simulink model "main"  (R2023a)
settings: Solver=VariableStepAuto  StartTime=0.0  StopTime=1  RelTol=1e-9  AbsTol=1e-9  EnableMultiTasking=on
values from neighbouring files (symbols this model uses):
  a_el = [r_ej,h_ej,r_ej]    [data.m]    (also in fo_python_to_matlab.m = [ax,ay,az])
  akt_GH = rand(1,13)*1    [inverse_dynamics.m]    (also in odvozeni_svaly.m = sym('akt_GH',[1 N_GH]))
  akt_ST = rand(1,13)*1    [inverse_dynamics.m]    (also in odvozeni_svaly.m = sym('akt_ST',[1 N_ST]))
  ax = r_ej    (= 0.088)    [data.m]
  ay = h_ej    (= 0.15)    [data.m]
  az = r_ej    (= 0.088)    [data.m]
  ccom = [-0.0110972, 0.00637508, 0.0541825]    [data.m]    (also in fo_python_to_matlab.m = [ccomx, ccomy, ccomz]; mm_python_to_matlab.m = [ccomx, ccomy, ccomz])
  cI = [5.75482e-05, 6.05521e-05, 1.05345e-05,-1.27405e-05, 1.65861e-05, 4.50136e-06]    [data.m]    (also in mm_python_to_matlab.m = [cixx, ciyy, cizz, cixy, ciyz, cizx])
  cont1 = [-0.083529 -0.01368 -0.098954]-scom    [data.m]    (also in fo_python_to_matlab.m = [x_cont1,y_cont1,z_cont1])
  cont2 = [-0.105456 -0.125076 -0.075251]-scom    [data.m]    (also in fo_python_to_matlab.m = [x_cont2,y_cont2,z_cont2])
  cont_params = [k_contact, eps]    [data.m]    (also in fo_python_to_matlab.m)
  Glenohumeral_F0M = str2double(table2array(GH(:,2)))'    [data.m]
  Glenohumeral_l0 = str2double(table2array(GH(:,3)))'    [data.m]
  h_ej = 0.15    [data.m]
  hcom = [0.000389382, -0.116338, -0.00231072]    [data.m]    (also in fo_python_to_matlab.m = [hcomx, hcomy, hcomz]; mm_python_to_matlab.m = [hcomx, hcomy, hcomz])
  hI = [0.00326632, 4.34807e-05, 0.00325004,-0.000136456, -1.30958e-06, -1.14964e-05]    [data.m]    (also in mm_python_to_matlab.m = [hixx, hiyy, hizz, hixy, hiyz, hizx])
  initialConditions = zeros(1,18)    [inverse_dynamics.m]
  k_contact = 0    [data.m]
  m = [0.0370005,0.12759,0.26363]    [data.m]    (also in fo_python_to_matlab.m = [c_m,s_m,h_m]; mm_python_to_matlab.m = [c_m,s_m,h_m])
  m_el = [x_ej,y_ej,z_ej]    [data.m]    (also in fo_python_to_matlab.m = [mx, my, mz])
  mx = x_ej    (= -0.03)    [data.m]
  my = y_ej    (= -0.1)    [data.m]
  mz = z_ej    (= 0.05)    [data.m]
  p = [c,k,g]    [data.m]    (also in fo_python_to_matlab.m)
  r_ej = 0.088    [data.m]
  Scapulothoracic_F0M = str2double(table2array(ST(:,2)))'    [data.m]
  Scapulothoracic_l0 = str2double(table2array(ST(:,3)))'    [data.m]
  scom = [-0.0512948, -0.0367122, -0.0430756]    [data.m]    (also in fo_python_to_matlab.m = [scomx, scomy, scomz]; mm_python_to_matlab.m = [scomx, scomy, scomz])
  sI = [0.00020065, 0.000202939, 0.000227237,-4.55661e-05, -7.53511e-05, -7.42694e-05]    [data.m]    (also in mm_python_to_matlab.m = [sixx, siyy, sizz, sixy, siyz, sizx])
  T_c = [-0.01433 0.02007 0.135535]    [data.m]    (also in fo_python_to_matlab.m = [T_cx,T_cy,T_cz]; mm_python_to_matlab.m = [T_cx,T_cy,T_cz]; odvozeni_svaly.m)
  T_d = 1e-20    [data.m]
  T_s = [-0.00955 -0.034 0.009]    [data.m]    (also in fo_python_to_matlab.m = [T_sx,T_sy,T_sz]; mm_python_to_matlab.m = [T_sx,T_sy,T_sz]; odvozeni_svaly.m)
  T_t = [0.006325 0.00693 0.025465]    [data.m]    (also in fo_python_to_matlab.m = [T_tx, T_ty, T_tz]; odvozeni_svaly.m)
  x_ej = -0.03    [data.m]
  y_ej = -0.1    [data.m]
  z_ej = 0.05    [data.m]
undefined symbols (not defined in the file or in its folder): phi_0, r_0, r_10, r_20, X, Y, Z
libraries: sm_lib x160, nesl_utility x89
(part 2 of 5)

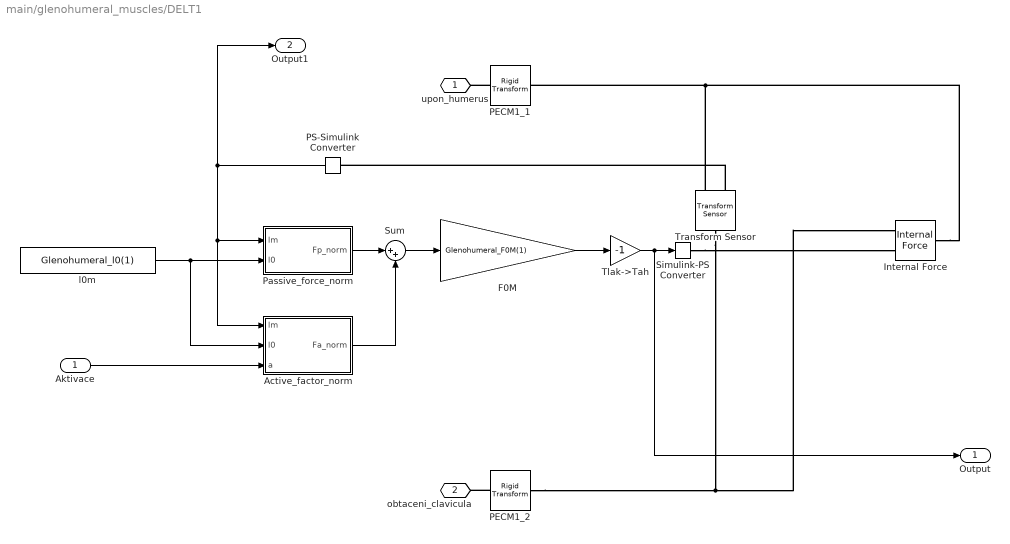
== system main/glenohumeral_muscles/DELT1 ==
  Aktivace : Inport
  Active_factor_norm : MATLAB Function  TreatAsAtomicUnit=on
  F0M : Gain  Gain=Glenohumeral_F0M(1)
  Internal Force : sm_lib/Forces and Torques/Internal Force
  PECM1_1 : sm_lib/Frames and Transforms/Rigid Transform  TranslationMethod=Cartesian  TranslationStandardOffset=0  TranslationStandardOffsetUnits=m  TranslationStandardAxis=+Z  TranslationCartesianOffset=[0.005 -0.104 0.008]  TranslationCartesianOffsetUnits=m  TranslationROffset=0  TranslationROffsetUnits=m  TranslationZOffset=0  TranslationZOffsetUnits=m  TranslationThetaOffset=0  TranslationThetaOffsetUnits=deg  RotationMethod=None  RotationAngleUnits=deg  RotationStandardAxis=+Z  RotationAngle=0.0  RotationArbitraryAxis=[0 0 1]  FollAlignAxisA=+X  BaseAlignAxisA=+Y  FollAlignAxisB=+Y  BaseAlignAxisB=+Z  RotationSequenceAxes=FollowerAxes  RotationSequence=XYX  RotationSequenceAngles=[0 0 0]  RotationSequenceAnglesUnits=deg  RotationMatrix=[1 0 0; 0 1 0; 0 0 1]  Quaternion=[1 0 0 0]
  PECM1_2 : sm_lib/Frames and Transforms/Rigid Transform  TranslationMethod=Cartesian  TranslationStandardOffset=0  TranslationStandardOffsetUnits=m  TranslationStandardAxis=+Z  TranslationCartesianOffset=[-0.002 0.032 0.131]  TranslationCartesianOffsetUnits=m  TranslationROffset=0  TranslationROffsetUnits=m  TranslationZOffset=0  TranslationZOffsetUnits=m  TranslationThetaOffset=0  TranslationThetaOffsetUnits=deg  RotationMethod=None  RotationAngleUnits=deg  RotationStandardAxis=+Y  RotationAngle=90  RotationArbitraryAxis=[0 0 1]  FollAlignAxisA=+X  BaseAlignAxisA=+Y  FollAlignAxisB=+Y  BaseAlignAxisB=+Z  RotationSequenceAxes=FollowerAxes  RotationSequence=XYX  RotationSequenceAngles=[0 0 0]  RotationSequenceAnglesUnits=deg  RotationMatrix=[1 0 0; 0 1 0; 0 0 1]  Quaternion=[1 0 0 0]
  PS-Simulink Converter : nesl_utility/PS-Simulink Converter  PhysicalDomain=network_engine_domain  SubClassName=ps_output  LeftPortType=input  RightPortType=output  PseudoPeriodic=off  Frequencies=[]  VectorFormat=inherit  Unit=inherit  AffineConversion=off
  Passive_force_norm : MATLAB Function  TreatAsAtomicUnit=on
  Simulink-PS Converter : nesl_utility/Simulink-PS Converter  PhysicalDomain=network_engine_domain  SubClassName=ps_input  LeftPortType=input  RightPortType=output  PseudoPeriodic=off  Frequencies=[]  NoiseDistribution=none  NoiseParameters=[]  Unit=1  AffineConversion=off  FilteringAndDerivatives=provide  SimscapeFilterOrder=1  InputFilterTimeConstant=0.001  UdotUserProvided=0
  Sum : Sum  Inputs=|++
  Tlak->Tah : Gain  Gain=-1
  Transform Sensor : sm_lib/Frames and Transforms/Transform Sensor  MeasurementFrame=World  RotationSequence=XYX  SenseAngle=off  SenseAxis=off  SenseQ=off  SenseR=off  SenseRotationSequence=off  SenseOmegaX=off  SenseOmegaY=off  SenseOmegaZ=off  SenseQDot=off  SenseRDot=off  SenseRotationSequenceDot=off  SenseAlphaX=off  SenseAlphaY=off  SenseAlphaZ=off  SenseQDDot=off  SenseRDDot=off  SenseX=off  SenseY=off  SenseZ=off  SenseRad=off  SenseAzim=off  SenseDist=on  SenseInc=off  SenseXDot=off  SenseYDot=off  SenseZDot=off  SenseRadDot=off  SenseAzimDot=off  SenseDistDot=off  SenseIncDot=off  SenseXDDot=off  SenseYDDot=off  SenseZDDot=off  SenseRadDDot=off  SenseAzimDDot=off  SenseDistDDot=off  SenseIncDDot=off
  l0m : Constant  Value=Glenohumeral_l0(1)
  upon_humerus : PMIOPort  Side=Left
  obtaceni_clavicula : PMIOPort  Port=2  Side=Left
  Output : Outport
  Output1 : Outport  Port=2
  wires:
  Sum/1 -> F0M/1
  F0M/1 -> Tlak->Tah/1
  Passive_force_norm/1(Fp_norm) -> Sum/1
  Active_factor_norm/1(Fa_norm) -> Sum/2
  Tlak->Tah/1 -> Output/1, Simulink-PS Converter/1
  PS-Simulink Converter/1 -> Output1/1, Active_factor_norm/1(lm), Passive_force_norm/1(lm)
  l0m/1 -> Active_factor_norm/2(l0), Passive_force_norm/2(l0)
  Aktivace/1 -> Active_factor_norm/3(a)
  connections:
  PECM1_2/RConn1 -- Internal Force/LConn1 -- Transform Sensor/LConn1
  PECM1_1/LConn1 -- upon_humerus/RConn1
  Internal Force/RConn1 -- Transform Sensor/RConn1 -- PECM1_1/RConn1
  PECM1_2/LConn1 -- obtaceni_clavicula/RConn1
  Simulink-PS Converter/RConn1 -- Internal Force/LConn2
  Transform Sensor/RConn2 -- PS-Simulink Converter/LConn1

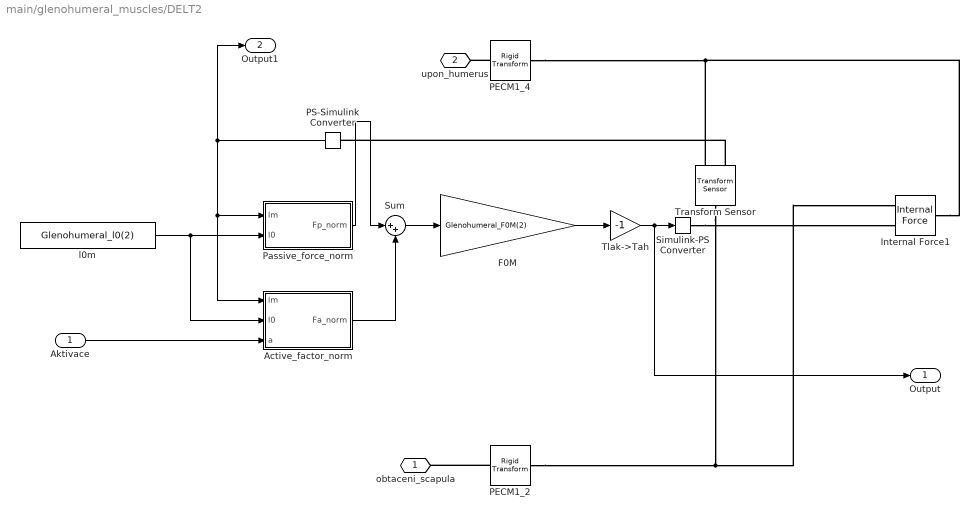
== system main/glenohumeral_muscles/DELT2 ==
  Aktivace : Inport
  Active_factor_norm : MATLAB Function  TreatAsAtomicUnit=on
  F0M : Gain  Gain=Glenohumeral_F0M(2)
  Internal Force1 : sm_lib/Forces and Torques/Internal Force
  PECM1_2 : sm_lib/Frames and Transforms/Rigid Transform  TranslationMethod=Cartesian  TranslationStandardOffset=0  TranslationStandardOffsetUnits=m  TranslationStandardAxis=+Z  TranslationCartesianOffset=[-0.028 -0.005 0.025]  TranslationCartesianOffsetUnits=m  TranslationROffset=0  TranslationROffsetUnits=m  TranslationZOffset=0  TranslationZOffsetUnits=m  TranslationThetaOffset=0  TranslationThetaOffsetUnits=deg  RotationMethod=None  RotationAngleUnits=deg  RotationStandardAxis=+Z  RotationAngle=0.0  RotationArbitraryAxis=[0 0 1]  FollAlignAxisA=+X  BaseAlignAxisA=+Y  FollAlignAxisB=+Y  BaseAlignAxisB=+Z  RotationSequenceAxes=FollowerAxes  RotationSequence=XYX  RotationSequenceAngles=[0 0 0]  RotationSequenceAnglesUnits=deg  RotationMatrix=[1 0 0; 0 1 0; 0 0 1]  Quaternion=[1 0 0 0]
  PECM1_4 : sm_lib/Frames and Transforms/Rigid Transform  TranslationMethod=Cartesian  TranslationStandardOffset=0  TranslationStandardOffsetUnits=m  TranslationStandardAxis=+Z  TranslationCartesianOffset=[-0.004 -0.058 0.028]  TranslationCartesianOffsetUnits=m  TranslationROffset=0  TranslationROffsetUnits=m  TranslationZOffset=0  TranslationZOffsetUnits=m  TranslationThetaOffset=0  TranslationThetaOffsetUnits=deg  RotationMethod=StandardAxis  RotationAngleUnits=deg  RotationStandardAxis=+Y  RotationAngle=90  RotationArbitraryAxis=[0 0 1]  FollAlignAxisA=+X  BaseAlignAxisA=+Y  FollAlignAxisB=+Y  BaseAlignAxisB=+Z  RotationSequenceAxes=FollowerAxes  RotationSequence=XYX  RotationSequenceAngles=[0 0 0]  RotationSequenceAnglesUnits=deg  RotationMatrix=[1 0 0; 0 1 0; 0 0 1]  Quaternion=[1 0 0 0]
  PS-Simulink Converter : nesl_utility/PS-Simulink Converter  PhysicalDomain=network_engine_domain  SubClassName=ps_output  LeftPortType=input  RightPortType=output  PseudoPeriodic=off  Frequencies=[]  VectorFormat=inherit  Unit=inherit  AffineConversion=off
  Passive_force_norm : MATLAB Function  TreatAsAtomicUnit=on
  Simulink-PS Converter : nesl_utility/Simulink-PS Converter  PhysicalDomain=network_engine_domain  SubClassName=ps_input  LeftPortType=input  RightPortType=output  PseudoPeriodic=off  Frequencies=[]  NoiseDistribution=none  NoiseParameters=[]  Unit=1  AffineConversion=off  FilteringAndDerivatives=provide  SimscapeFilterOrder=1  InputFilterTimeConstant=0.001  UdotUserProvided=0
  Sum : Sum  Inputs=|++
  Tlak->Tah : Gain  Gain=-1
  Transform Sensor : sm_lib/Frames and Transforms/Transform Sensor  MeasurementFrame=World  RotationSequence=XYX  SenseAngle=off  SenseAxis=off  SenseQ=off  SenseR=off  SenseRotationSequence=off  SenseOmegaX=off  SenseOmegaY=off  SenseOmegaZ=off  SenseQDot=off  SenseRDot=off  SenseRotationSequenceDot=off  SenseAlphaX=off  SenseAlphaY=off  SenseAlphaZ=off  SenseQDDot=off  SenseRDDot=off  SenseX=off  SenseY=off  SenseZ=off  SenseRad=off  SenseAzim=off  SenseDist=on  SenseInc=off  SenseXDot=off  SenseYDot=off  SenseZDot=off  SenseRadDot=off  SenseAzimDot=off  SenseDistDot=off  SenseIncDot=off  SenseXDDot=off  SenseYDDot=off  SenseZDDot=off  SenseRadDDot=off  SenseAzimDDot=off  SenseDistDDot=off  SenseIncDDot=off
  l0m : Constant  Value=Glenohumeral_l0(2)
  obtaceni_scapula : PMIOPort  Side=Left
  upon_humerus : PMIOPort  Port=2  Side=Left
  Output : Outport
  Output1 : Outport  Port=2
  wires:
  Passive_force_norm/1(Fp_norm) -> Sum/1
  F0M/1 -> Tlak->Tah/1
  Sum/1 -> F0M/1
  Active_factor_norm/1(Fa_norm) -> Sum/2
  Tlak->Tah/1 -> Output/1, Simulink-PS Converter/1
  PS-Simulink Converter/1 -> Output1/1, Active_factor_norm/1(lm), Passive_force_norm/1(lm)
  l0m/1 -> Active_factor_norm/2(l0), Passive_force_norm/2(l0)
  Aktivace/1 -> Active_factor_norm/3(a)
  connections:
  Transform Sensor/LConn1 -- PECM1_2/RConn1 -- Internal Force1/LConn1
  Transform Sensor/RConn1 -- PECM1_4/RConn1 -- Internal Force1/RConn1
  PECM1_2/LConn1 -- obtaceni_scapula/RConn1
  PECM1_4/LConn1 -- upon_humerus/RConn1
  Simulink-PS Converter/RConn1 -- Internal Force1/LConn2
  Transform Sensor/RConn2 -- PS-Simulink Converter/LConn1

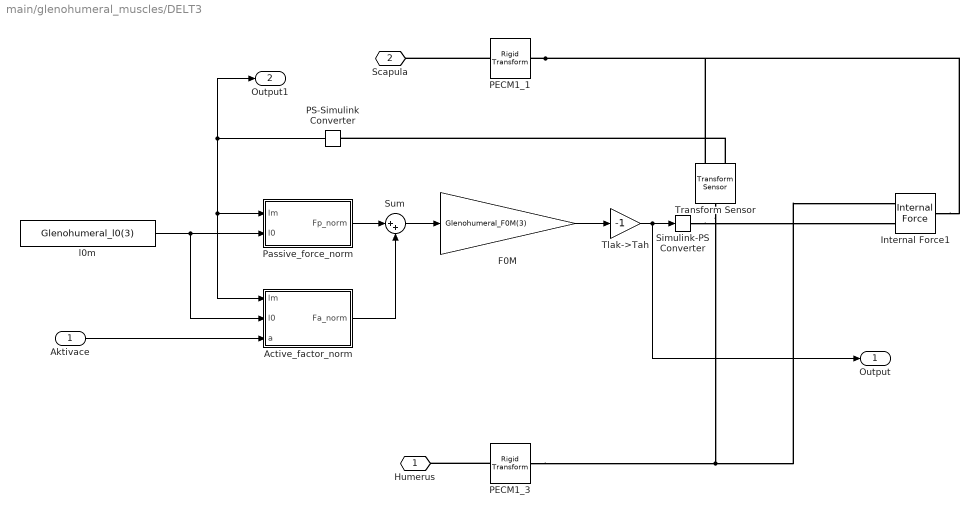
== system main/glenohumeral_muscles/DELT3 ==
  Aktivace : Inport
  Active_factor_norm : MATLAB Function  TreatAsAtomicUnit=on
  F0M : Gain  Gain=Glenohumeral_F0M(3)
  Internal Force1 : sm_lib/Forces and Torques/Internal Force
  PECM1_1 : sm_lib/Frames and Transforms/Rigid Transform  TranslationMethod=Cartesian  TranslationStandardOffset=0  TranslationStandardOffsetUnits=m  TranslationStandardAxis=+Z  TranslationCartesianOffset=[-0.072 -0.024 0.006]  TranslationCartesianOffsetUnits=m  TranslationROffset=0  TranslationROffsetUnits=m  TranslationZOffset=0  TranslationZOffsetUnits=m  TranslationThetaOffset=0  TranslationThetaOffsetUnits=deg  RotationMethod=None  RotationAngleUnits=deg  RotationStandardAxis=+Z  RotationAngle=0.0  RotationArbitraryAxis=[0 0 1]  FollAlignAxisA=+X  BaseAlignAxisA=+Y  FollAlignAxisB=+Y  BaseAlignAxisB=+Z  RotationSequenceAxes=FollowerAxes  RotationSequence=XYX  RotationSequenceAngles=[0 0 0]  RotationSequenceAnglesUnits=deg  RotationMatrix=[1 0 0; 0 1 0; 0 0 1]  Quaternion=[1 0 0 0]
  PECM1_3 : sm_lib/Frames and Transforms/Rigid Transform  TranslationMethod=Cartesian  TranslationStandardOffset=0  TranslationStandardOffsetUnits=m  TranslationStandardAxis=+Z  TranslationCartesianOffset=[-0.019 -0.05 0.006]  TranslationCartesianOffsetUnits=m  TranslationROffset=0  TranslationROffsetUnits=m  TranslationZOffset=0  TranslationZOffsetUnits=m  TranslationThetaOffset=0  TranslationThetaOffsetUnits=deg  RotationMethod=StandardAxis  RotationAngleUnits=deg  RotationStandardAxis=+Y  RotationAngle=90  RotationArbitraryAxis=[0 0 1]  FollAlignAxisA=+X  BaseAlignAxisA=+Y  FollAlignAxisB=+Y  BaseAlignAxisB=+Z  RotationSequenceAxes=FollowerAxes  RotationSequence=XYX  RotationSequenceAngles=[0 0 0]  RotationSequenceAnglesUnits=deg  RotationMatrix=[1 0 0; 0 1 0; 0 0 1]  Quaternion=[1 0 0 0]
  PS-Simulink Converter : nesl_utility/PS-Simulink Converter  PhysicalDomain=network_engine_domain  SubClassName=ps_output  LeftPortType=input  RightPortType=output  PseudoPeriodic=off  Frequencies=[]  VectorFormat=inherit  Unit=inherit  AffineConversion=off
  Passive_force_norm : MATLAB Function  TreatAsAtomicUnit=on
  Simulink-PS Converter : nesl_utility/Simulink-PS Converter  PhysicalDomain=network_engine_domain  SubClassName=ps_input  LeftPortType=input  RightPortType=output  PseudoPeriodic=off  Frequencies=[]  NoiseDistribution=none  NoiseParameters=[]  Unit=1  AffineConversion=off  FilteringAndDerivatives=provide  SimscapeFilterOrder=1  InputFilterTimeConstant=0.001  UdotUserProvided=0
  Sum : Sum  Inputs=|++
  Tlak->Tah : Gain  Gain=-1
  Transform Sensor : sm_lib/Frames and Transforms/Transform Sensor  MeasurementFrame=World  RotationSequence=XYX  SenseAngle=off  SenseAxis=off  SenseQ=off  SenseR=off  SenseRotationSequence=off  SenseOmegaX=off  SenseOmegaY=off  SenseOmegaZ=off  SenseQDot=off  SenseRDot=off  SenseRotationSequenceDot=off  SenseAlphaX=off  SenseAlphaY=off  SenseAlphaZ=off  SenseQDDot=off  SenseRDDot=off  SenseX=off  SenseY=off  SenseZ=off  SenseRad=off  SenseAzim=off  SenseDist=on  SenseInc=off  SenseXDot=off  SenseYDot=off  SenseZDot=off  SenseRadDot=off  SenseAzimDot=off  SenseDistDot=off  SenseIncDot=off  SenseXDDot=off  SenseYDDot=off  SenseZDDot=off  SenseRadDDot=off  SenseAzimDDot=off  SenseDistDDot=off  SenseIncDDot=off
  l0m : Constant  Value=Glenohumeral_l0(3)
  Humerus : PMIOPort  Side=Left
  Scapula : PMIOPort  Port=2  Side=Left
  Output : Outport
  Output1 : Outport  Port=2
  wires:
  l0m/1 -> Active_factor_norm/2(l0), Passive_force_norm/2(l0)
  Tlak->Tah/1 -> Output/1, Simulink-PS Converter/1
  PS-Simulink Converter/1 -> Output1/1, Active_factor_norm/1(lm), Passive_force_norm/1(lm)
  Active_factor_norm/1(Fa_norm) -> Sum/2
  Sum/1 -> F0M/1
  Passive_force_norm/1(Fp_norm) -> Sum/1
  F0M/1 -> Tlak->Tah/1
  Aktivace/1 -> Active_factor_norm/3(a)
  connections:
  PECM1_1/RConn1 -- Internal Force1/RConn1 -- Transform Sensor/RConn1
  PECM1_3/RConn1 -- Internal Force1/LConn1 -- Transform Sensor/LConn1
  Transform Sensor/RConn2 -- PS-Simulink Converter/LConn1
  Simulink-PS Converter/RConn1 -- Internal Force1/LConn2
  PECM1_3/LConn1 -- Humerus/RConn1
  PECM1_1/LConn1 -- Scapula/RConn1

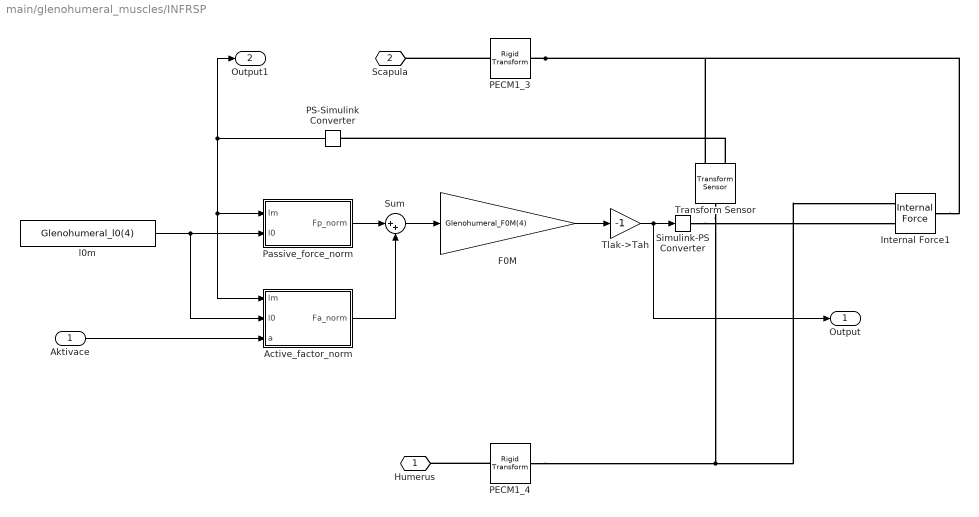
== system main/glenohumeral_muscles/INFRSP ==
  Aktivace : Inport
  Active_factor_norm : MATLAB Function  TreatAsAtomicUnit=on
  F0M : Gain  Gain=Glenohumeral_F0M(4)
  Internal Force1 : sm_lib/Forces and Torques/Internal Force
  PECM1_3 : sm_lib/Frames and Transforms/Rigid Transform  TranslationMethod=Cartesian  TranslationStandardOffset=0  TranslationStandardOffsetUnits=m  TranslationStandardAxis=+Z  TranslationCartesianOffset=[-0.043 -0.048 -0.022]  TranslationCartesianOffsetUnits=m  TranslationROffset=0  TranslationROffsetUnits=m  TranslationZOffset=0  TranslationZOffsetUnits=m  TranslationThetaOffset=0  TranslationThetaOffsetUnits=deg  RotationMethod=None  RotationAngleUnits=deg  RotationStandardAxis=+Z  RotationAngle=0.0  RotationArbitraryAxis=[0 0 1]  FollAlignAxisA=+X  BaseAlignAxisA=+Y  FollAlignAxisB=+Y  BaseAlignAxisB=+Z  RotationSequenceAxes=FollowerAxes  RotationSequence=XYX  RotationSequenceAngles=[0 0 0]  RotationSequenceAnglesUnits=deg  RotationMatrix=[1 0 0; 0 1 0; 0 0 1]  Quaternion=[1 0 0 0]
  PECM1_4 : sm_lib/Frames and Transforms/Rigid Transform  TranslationMethod=Cartesian  TranslationStandardOffset=0  TranslationStandardOffsetUnits=m  TranslationStandardAxis=+Z  TranslationCartesianOffset=[-0.005 0.008 0.026]  TranslationCartesianOffsetUnits=m  TranslationROffset=0  TranslationROffsetUnits=m  TranslationZOffset=0  TranslationZOffsetUnits=m  TranslationThetaOffset=0  TranslationThetaOffsetUnits=deg  RotationMethod=StandardAxis  RotationAngleUnits=deg  RotationStandardAxis=+Y  RotationAngle=90  RotationArbitraryAxis=[0 0 1]  FollAlignAxisA=+X  BaseAlignAxisA=+Y  FollAlignAxisB=+Y  BaseAlignAxisB=+Z  RotationSequenceAxes=FollowerAxes  RotationSequence=XYX  RotationSequenceAngles=[0 0 0]  RotationSequenceAnglesUnits=deg  RotationMatrix=[1 0 0; 0 1 0; 0 0 1]  Quaternion=[1 0 0 0]
  PS-Simulink Converter : nesl_utility/PS-Simulink Converter  PhysicalDomain=network_engine_domain  SubClassName=ps_output  LeftPortType=input  RightPortType=output  PseudoPeriodic=off  Frequencies=[]  VectorFormat=inherit  Unit=inherit  AffineConversion=off
  Passive_force_norm : MATLAB Function  TreatAsAtomicUnit=on
  Simulink-PS Converter : nesl_utility/Simulink-PS Converter  PhysicalDomain=network_engine_domain  SubClassName=ps_input  LeftPortType=input  RightPortType=output  PseudoPeriodic=off  Frequencies=[]  NoiseDistribution=none  NoiseParameters=[]  Unit=1  AffineConversion=off  FilteringAndDerivatives=provide  SimscapeFilterOrder=1  InputFilterTimeConstant=0.001  UdotUserProvided=0
  Sum : Sum  Inputs=|++
  Tlak->Tah : Gain  Gain=-1
  Transform Sensor : sm_lib/Frames and Transforms/Transform Sensor  MeasurementFrame=World  RotationSequence=XYX  SenseAngle=off  SenseAxis=off  SenseQ=off  SenseR=off  SenseRotationSequence=off  SenseOmegaX=off  SenseOmegaY=off  SenseOmegaZ=off  SenseQDot=off  SenseRDot=off  SenseRotationSequenceDot=off  SenseAlphaX=off  SenseAlphaY=off  SenseAlphaZ=off  SenseQDDot=off  SenseRDDot=off  SenseX=off  SenseY=off  SenseZ=off  SenseRad=off  SenseAzim=off  SenseDist=on  SenseInc=off  SenseXDot=off  SenseYDot=off  SenseZDot=off  SenseRadDot=off  SenseAzimDot=off  SenseDistDot=off  SenseIncDot=off  SenseXDDot=off  SenseYDDot=off  SenseZDDot=off  SenseRadDDot=off  SenseAzimDDot=off  SenseDistDDot=off  SenseIncDDot=off
  l0m : Constant  Value=Glenohumeral_l0(4)
  Humerus : PMIOPort  Side=Left
  Scapula : PMIOPort  Port=2  Side=Left
  Output : Outport
  Output1 : Outport  Port=2
  wires:
  PS-Simulink Converter/1 -> Output1/1, Active_factor_norm/1(lm), Passive_force_norm/1(lm)
  l0m/1 -> Active_factor_norm/2(l0), Passive_force_norm/2(l0)
  Tlak->Tah/1 -> Output/1, Simulink-PS Converter/1
  Sum/1 -> F0M/1
  F0M/1 -> Tlak->Tah/1
  Aktivace/1 -> Active_factor_norm/3(a)
  Passive_force_norm/1(Fp_norm) -> Sum/1
  Active_factor_norm/1(Fa_norm) -> Sum/2
  connections:
  PECM1_4/RConn1 -- Internal Force1/LConn1 -- Transform Sensor/LConn1
  PECM1_3/RConn1 -- Internal Force1/RConn1 -- Transform Sensor/RConn1
  PECM1_3/LConn1 -- Scapula/RConn1
  Simulink-PS Converter/RConn1 -- Internal Force1/LConn2
  PECM1_4/LConn1 -- Humerus/RConn1
  Transform Sensor/RConn2 -- PS-Simulink Converter/LConn1

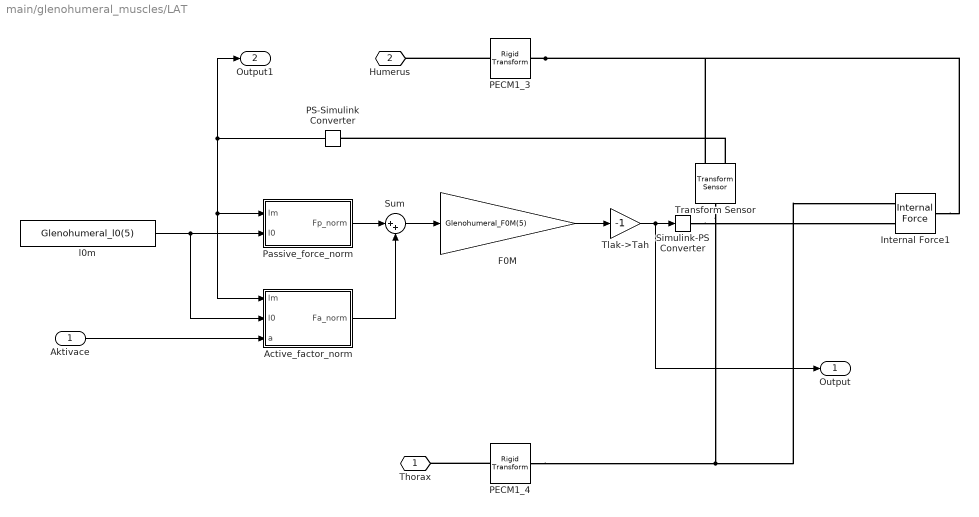
== system main/glenohumeral_muscles/LAT ==
  Aktivace : Inport
  Active_factor_norm : MATLAB Function  TreatAsAtomicUnit=on
  F0M : Gain  Gain=Glenohumeral_F0M(5)
  Internal Force1 : sm_lib/Forces and Torques/Internal Force
  PECM1_3 : sm_lib/Frames and Transforms/Rigid Transform  TranslationMethod=Cartesian  TranslationStandardOffset=0  TranslationStandardOffsetUnits=m  TranslationStandardAxis=+Z  TranslationCartesianOffset=[0.002 -0.019 -0.021]  TranslationCartesianOffsetUnits=m  TranslationROffset=0  TranslationROffsetUnits=m  TranslationZOffset=0  TranslationZOffsetUnits=m  TranslationThetaOffset=0  TranslationThetaOffsetUnits=deg  RotationMethod=None  RotationAngleUnits=deg  RotationStandardAxis=+Z  RotationAngle=0.0  RotationArbitraryAxis=[0 0 1]  FollAlignAxisA=+X  BaseAlignAxisA=+Y  FollAlignAxisB=+Y  BaseAlignAxisB=+Z  RotationSequenceAxes=FollowerAxes  RotationSequence=XYX  RotationSequenceAngles=[0 0 0]  RotationSequenceAnglesUnits=deg  RotationMatrix=[1 0 0; 0 1 0; 0 0 1]  Quaternion=[1 0 0 0]
  PECM1_4 : sm_lib/Frames and Transforms/Rigid Transform  TranslationMethod=Cartesian  TranslationStandardOffset=0  TranslationStandardOffsetUnits=m  TranslationStandardAxis=+Z  TranslationCartesianOffset=[-0.095 -0.161 0.001]  TranslationCartesianOffsetUnits=m  TranslationROffset=0  TranslationROffsetUnits=m  TranslationZOffset=0  TranslationZOffsetUnits=m  TranslationThetaOffset=0  TranslationThetaOffsetUnits=deg  RotationMethod=StandardAxis  RotationAngleUnits=deg  RotationStandardAxis=+Y  RotationAngle=90  RotationArbitraryAxis=[0 0 1]  FollAlignAxisA=+X  BaseAlignAxisA=+Y  FollAlignAxisB=+Y  BaseAlignAxisB=+Z  RotationSequenceAxes=FollowerAxes  RotationSequence=XYX  RotationSequenceAngles=[0 0 0]  RotationSequenceAnglesUnits=deg  RotationMatrix=[1 0 0; 0 1 0; 0 0 1]  Quaternion=[1 0 0 0]
  PS-Simulink Converter : nesl_utility/PS-Simulink Converter  PhysicalDomain=network_engine_domain  SubClassName=ps_output  LeftPortType=input  RightPortType=output  PseudoPeriodic=off  Frequencies=[]  VectorFormat=inherit  Unit=inherit  AffineConversion=off
  Passive_force_norm : MATLAB Function  TreatAsAtomicUnit=on
  Simulink-PS Converter : nesl_utility/Simulink-PS Converter  PhysicalDomain=network_engine_domain  SubClassName=ps_input  LeftPortType=input  RightPortType=output  PseudoPeriodic=off  Frequencies=[]  NoiseDistribution=none  NoiseParameters=[]  Unit=1  AffineConversion=off  FilteringAndDerivatives=provide  SimscapeFilterOrder=1  InputFilterTimeConstant=0.001  UdotUserProvided=0
  Sum : Sum  Inputs=|++
  Tlak->Tah : Gain  Gain=-1
  Transform Sensor : sm_lib/Frames and Transforms/Transform Sensor  MeasurementFrame=World  RotationSequence=XYX  SenseAngle=off  SenseAxis=off  SenseQ=off  SenseR=off  SenseRotationSequence=off  SenseOmegaX=off  SenseOmegaY=off  SenseOmegaZ=off  SenseQDot=off  SenseRDot=off  SenseRotationSequenceDot=off  SenseAlphaX=off  SenseAlphaY=off  SenseAlphaZ=off  SenseQDDot=off  SenseRDDot=off  SenseX=off  SenseY=off  SenseZ=off  SenseRad=off  SenseAzim=off  SenseDist=on  SenseInc=off  SenseXDot=off  SenseYDot=off  SenseZDot=off  SenseRadDot=off  SenseAzimDot=off  SenseDistDot=off  SenseIncDot=off  SenseXDDot=off  SenseYDDot=off  SenseZDDot=off  SenseRadDDot=off  SenseAzimDDot=off  SenseDistDDot=off  SenseIncDDot=off
  l0m : Constant  Value=Glenohumeral_l0(5)
  Thorax : PMIOPort  Side=Left
  Humerus : PMIOPort  Port=2  Side=Left
  Output : Outport
  Output1 : Outport  Port=2
  wires:
  Active_factor_norm/1(Fa_norm) -> Sum/2
  Passive_force_norm/1(Fp_norm) -> Sum/1
  Tlak->Tah/1 -> Output/1, Simulink-PS Converter/1
  Aktivace/1 -> Active_factor_norm/3(a)
  PS-Simulink Converter/1 -> Output1/1, Active_factor_norm/1(lm), Passive_force_norm/1(lm)
  F0M/1 -> Tlak->Tah/1
  l0m/1 -> Active_factor_norm/2(l0), Passive_force_norm/2(l0)
  Sum/1 -> F0M/1
  connections:
  PECM1_4/RConn1 -- Internal Force1/LConn1 -- Transform Sensor/LConn1
  PECM1_3/RConn1 -- Internal Force1/RConn1 -- Transform Sensor/RConn1
  PECM1_3/LConn1 -- Humerus/RConn1
  PECM1_4/LConn1 -- Thorax/RConn1
  Simulink-PS Converter/RConn1 -- Internal Force1/LConn2
  Transform Sensor/RConn2 -- PS-Simulink Converter/LConn1

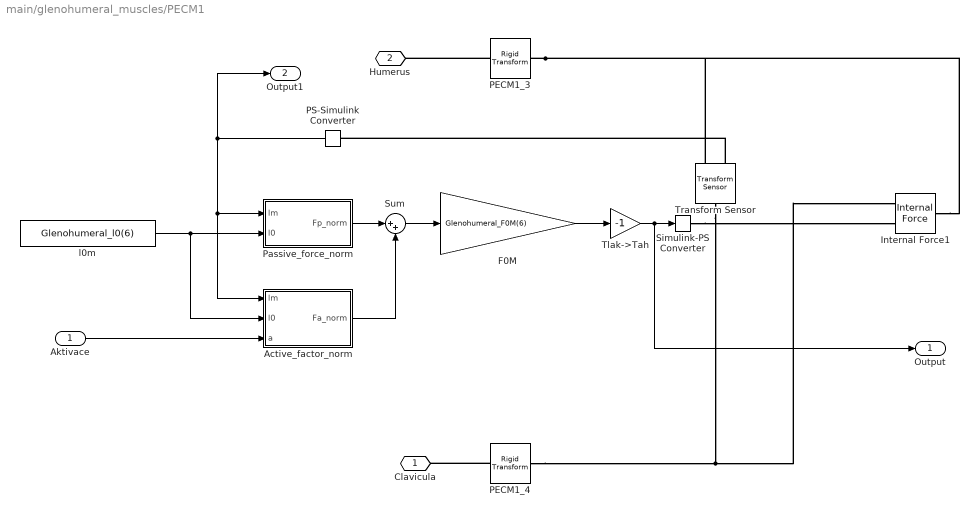
== system main/glenohumeral_muscles/PECM1 ==
  Aktivace : Inport
  Active_factor_norm : MATLAB Function  TreatAsAtomicUnit=on
  F0M : Gain  Gain=Glenohumeral_F0M(6)
  Internal Force1 : sm_lib/Forces and Torques/Internal Force
  PECM1_3 : sm_lib/Frames and Transforms/Rigid Transform  TranslationMethod=Cartesian  TranslationStandardOffset=0  TranslationStandardOffsetUnits=m  TranslationStandardAxis=+Z  TranslationCartesianOffset=[0.016 -0.04 0.005]  TranslationCartesianOffsetUnits=m  TranslationROffset=0  TranslationROffsetUnits=m  TranslationZOffset=0  TranslationZOffsetUnits=m  TranslationThetaOffset=0  TranslationThetaOffsetUnits=deg  RotationMethod=None  RotationAngleUnits=deg  RotationStandardAxis=+Z  RotationAngle=0.0  RotationArbitraryAxis=[0 0 1]  FollAlignAxisA=+X  BaseAlignAxisA=+Y  FollAlignAxisB=+Y  BaseAlignAxisB=+Z  RotationSequenceAxes=FollowerAxes  RotationSequence=XYX  RotationSequenceAngles=[0 0 0]  RotationSequenceAnglesUnits=deg  RotationMatrix=[1 0 0; 0 1 0; 0 0 1]  Quaternion=[1 0 0 0]
  PECM1_4 : sm_lib/Frames and Transforms/Rigid Transform  TranslationMethod=Cartesian  TranslationStandardOffset=0  TranslationStandardOffsetUnits=m  TranslationStandardAxis=+Z  TranslationCartesianOffset=[0 0.006 0.059]  TranslationCartesianOffsetUnits=m  TranslationROffset=0  TranslationROffsetUnits=m  TranslationZOffset=0  TranslationZOffsetUnits=m  TranslationThetaOffset=0  TranslationThetaOffsetUnits=deg  RotationMethod=StandardAxis  RotationAngleUnits=deg  RotationStandardAxis=+Y  RotationAngle=90  RotationArbitraryAxis=[0 0 1]  FollAlignAxisA=+X  BaseAlignAxisA=+Y  FollAlignAxisB=+Y  BaseAlignAxisB=+Z  RotationSequenceAxes=FollowerAxes  RotationSequence=XYX  RotationSequenceAngles=[0 0 0]  RotationSequenceAnglesUnits=deg  RotationMatrix=[1 0 0; 0 1 0; 0 0 1]  Quaternion=[1 0 0 0]
  PS-Simulink Converter : nesl_utility/PS-Simulink Converter  PhysicalDomain=network_engine_domain  SubClassName=ps_output  LeftPortType=input  RightPortType=output  PseudoPeriodic=off  Frequencies=[]  VectorFormat=inherit  Unit=inherit  AffineConversion=off
  Passive_force_norm : MATLAB Function  TreatAsAtomicUnit=on
  Simulink-PS Converter : nesl_utility/Simulink-PS Converter  PhysicalDomain=network_engine_domain  SubClassName=ps_input  LeftPortType=input  RightPortType=output  PseudoPeriodic=off  Frequencies=[]  NoiseDistribution=none  NoiseParameters=[]  Unit=1  AffineConversion=off  FilteringAndDerivatives=provide  SimscapeFilterOrder=1  InputFilterTimeConstant=0.001  UdotUserProvided=0
  Sum : Sum  Inputs=|++
  Tlak->Tah : Gain  Gain=-1
  Transform Sensor : sm_lib/Frames and Transforms/Transform Sensor  MeasurementFrame=World  RotationSequence=XYX  SenseAngle=off  SenseAxis=off  SenseQ=off  SenseR=off  SenseRotationSequence=off  SenseOmegaX=off  SenseOmegaY=off  SenseOmegaZ=off  SenseQDot=off  SenseRDot=off  SenseRotationSequenceDot=off  SenseAlphaX=off  SenseAlphaY=off  SenseAlphaZ=off  SenseQDDot=off  SenseRDDot=off  SenseX=off  SenseY=off  SenseZ=off  SenseRad=off  SenseAzim=off  SenseDist=on  SenseInc=off  SenseXDot=off  SenseYDot=off  SenseZDot=off  SenseRadDot=off  SenseAzimDot=off  SenseDistDot=off  SenseIncDot=off  SenseXDDot=off  SenseYDDot=off  SenseZDDot=off  SenseRadDDot=off  SenseAzimDDot=off  SenseDistDDot=off  SenseIncDDot=off
  l0m : Constant  Value=Glenohumeral_l0(6)
  Clavicula : PMIOPort  Side=Left
  Humerus : PMIOPort  Port=2  Side=Left
  Output : Outport
  Output1 : Outport  Port=2
  wires:
  Tlak->Tah/1 -> Output/1, Simulink-PS Converter/1
  l0m/1 -> Active_factor_norm/2(l0), Passive_force_norm/2(l0)
  Passive_force_norm/1(Fp_norm) -> Sum/1
  F0M/1 -> Tlak->Tah/1
  Aktivace/1 -> Active_factor_norm/3(a)
  Sum/1 -> F0M/1
  Active_factor_norm/1(Fa_norm) -> Sum/2
  PS-Simulink Converter/1 -> Output1/1, Active_factor_norm/1(lm), Passive_force_norm/1(lm)
  connections:
  PECM1_3/RConn1 -- Internal Force1/RConn1 -- Transform Sensor/RConn1
  PECM1_4/RConn1 -- Internal Force1/LConn1 -- Transform Sensor/LConn1
  PECM1_3/LConn1 -- Humerus/RConn1
  PECM1_4/LConn1 -- Clavicula/RConn1
  Transform Sensor/RConn2 -- PS-Simulink Converter/LConn1
  Simulink-PS Converter/RConn1 -- Internal Force1/LConn2

== system main/glenohumeral_muscles/PECM2 ==
  Aktivace : Inport
  Active_factor_norm : MATLAB Function  TreatAsAtomicUnit=on
  F0M : Gain  Gain=Glenohumeral_F0M(7)
  Internal Force1 : sm_lib/Forces and Torques/Internal Force
  PECM1_3 : sm_lib/Frames and Transforms/Rigid Transform  TranslationMethod=Cartesian  TranslationStandardOffset=0  TranslationStandardOffsetUnits=m  TranslationStandardAxis=+Z  TranslationCartesianOffset=[0.016 -0.035 0.005]  TranslationCartesianOffsetUnits=m  TranslationROffset=0  TranslationROffsetUnits=m  TranslationZOffset=0  TranslationZOffsetUnits=m  TranslationThetaOffset=0  TranslationThetaOffsetUnits=deg  RotationMethod=None  RotationAngleUnits=deg  RotationStandardAxis=+Z  RotationAngle=0.0  RotationArbitraryAxis=[0 0 1]  FollAlignAxisA=+X  BaseAlignAxisA=+Y  FollAlignAxisB=+Y  BaseAlignAxisB=+Z  RotationSequenceAxes=FollowerAxes  RotationSequence=XYX  RotationSequenceAngles=[0 0 0]  RotationSequenceAnglesUnits=deg  RotationMatrix=[1 0 0; 0 1 0; 0 0 1]  Quaternion=[1 0 0 0]
  PECM1_4 : sm_lib/Frames and Transforms/Rigid Transform  TranslationMethod=Cartesian  TranslationStandardOffset=0  TranslationStandardOffsetUnits=m  TranslationStandardAxis=+Z  TranslationCartesianOffset=[0.042 -0.043 0.081]  TranslationCartesianOffsetUnits=m  TranslationROffset=0  TranslationROffsetUnits=m  TranslationZOffset=0  TranslationZOffsetUnits=m  TranslationThetaOffset=0  TranslationThetaOffsetUnits=deg  RotationMethod=StandardAxis  RotationAngleUnits=deg  RotationStandardAxis=+Y  RotationAngle=90  RotationArbitraryAxis=[0 0 1]  FollAlignAxisA=+X  BaseAlignAxisA=+Y  FollAlignAxisB=+Y  BaseAlignAxisB=+Z  RotationSequenceAxes=FollowerAxes  RotationSequence=XYX  RotationSequenceAngles=[0 0 0]  RotationSequenceAnglesUnits=deg  RotationMatrix=[1 0 0; 0 1 0; 0 0 1]  Quaternion=[1 0 0 0]
  PS-Simulink Converter : nesl_utility/PS-Simulink Converter  PhysicalDomain=network_engine_domain  SubClassName=ps_output  LeftPortType=input  RightPortType=output  PseudoPeriodic=off  Frequencies=[]  VectorFormat=inherit  Unit=inherit  AffineConversion=off
  Passive_force_norm : MATLAB Function  TreatAsAtomicUnit=on
  Simulink-PS Converter : nesl_utility/Simulink-PS Converter  PhysicalDomain=network_engine_domain  SubClassName=ps_input  LeftPortType=input  RightPortType=output  PseudoPeriodic=off  Frequencies=[]  NoiseDistribution=none  NoiseParameters=[]  Unit=1  AffineConversion=off  FilteringAndDerivatives=provide  SimscapeFilterOrder=1  InputFilterTimeConstant=0.001  UdotUserProvided=0
  Sum : Sum  Inputs=|++
  Tlak->Tah : Gain  Gain=-1
  Transform Sensor : sm_lib/Frames and Transforms/Transform Sensor  MeasurementFrame=World  RotationSequence=XYX  SenseAngle=off  SenseAxis=off  SenseQ=off  SenseR=off  SenseRotationSequence=off  SenseOmegaX=off  SenseOmegaY=off  SenseOmegaZ=off  SenseQDot=off  SenseRDot=off  SenseRotationSequenceDot=off  SenseAlphaX=off  SenseAlphaY=off  SenseAlphaZ=off  SenseQDDot=off  SenseRDDot=off  SenseX=off  SenseY=off  SenseZ=off  SenseRad=off  SenseAzim=off  SenseDist=on  SenseInc=off  SenseXDot=off  SenseYDot=off  SenseZDot=off  SenseRadDot=off  SenseAzimDot=off  SenseDistDot=off  SenseIncDot=off  SenseXDDot=off  SenseYDDot=off  SenseZDDot=off  SenseRadDDot=off  SenseAzimDDot=off  SenseDistDDot=off  SenseIncDDot=off
  l0m : Constant  Value=Glenohumeral_l0(7)
  Thorax : PMIOPort  Side=Left
  Humerus : PMIOPort  Port=2  Side=Left
  Output : Outport
  Output1 : Outport  Port=2
  wires:
  l0m/1 -> Active_factor_norm/2(l0), Passive_force_norm/2(l0)
  Tlak->Tah/1 -> Output/1, Simulink-PS Converter/1
  PS-Simulink Converter/1 -> Output1/1, Active_factor_norm/1(lm), Passive_force_norm/1(lm)
  Aktivace/1 -> Active_factor_norm/3(a)
  Sum/1 -> F0M/1
  Active_factor_norm/1(Fa_norm) -> Sum/2
  Passive_force_norm/1(Fp_norm) -> Sum/1
  F0M/1 -> Tlak->Tah/1
  connections:
  PECM1_3/RConn1 -- Internal Force1/RConn1 -- Transform Sensor/RConn1
  PECM1_4/RConn1 -- Internal Force1/LConn1 -- Transform Sensor/LConn1
  PECM1_3/LConn1 -- Humerus/RConn1
  PECM1_4/LConn1 -- Thorax/RConn1
  Simulink-PS Converter/RConn1 -- Internal Force1/LConn2
  Transform Sensor/RConn2 -- PS-Simulink Converter/LConn1

== system main/glenohumeral_muscles/PECM3 ==
  Aktivace : Inport
  Active_factor_norm : MATLAB Function  TreatAsAtomicUnit=on
  F0M : Gain  Gain=Glenohumeral_F0M(8)
  Internal Force1 : sm_lib/Forces and Torques/Internal Force
  PECM1_3 : sm_lib/Frames and Transforms/Rigid Transform  TranslationMethod=Cartesian  TranslationStandardOffset=0  TranslationStandardOffsetUnits=m  TranslationStandardAxis=+Z  TranslationCartesianOffset=[0.016 -0.03 0.005]  TranslationCartesianOffsetUnits=m  TranslationROffset=0  TranslationROffsetUnits=m  TranslationZOffset=0  TranslationZOffsetUnits=m  TranslationThetaOffset=0  TranslationThetaOffsetUnits=deg  RotationMethod=None  RotationAngleUnits=deg  RotationStandardAxis=+Z  RotationAngle=0.0  RotationArbitraryAxis=[0 0 1]  FollAlignAxisA=+X  BaseAlignAxisA=+Y  FollAlignAxisB=+Y  BaseAlignAxisB=+Z  RotationSequenceAxes=FollowerAxes  RotationSequence=XYX  RotationSequenceAngles=[0 0 0]  RotationSequenceAnglesUnits=deg  RotationMatrix=[1 0 0; 0 1 0; 0 0 1]  Quaternion=[1 0 0 0]
  PECM1_4 : sm_lib/Frames and Transforms/Rigid Transform  TranslationMethod=Cartesian  TranslationStandardOffset=0  TranslationStandardOffsetUnits=m  TranslationStandardAxis=+Z  TranslationCartesianOffset=[0.043 -0.093 0.083]  TranslationCartesianOffsetUnits=m  TranslationROffset=0  TranslationROffsetUnits=m  TranslationZOffset=0  TranslationZOffsetUnits=m  TranslationThetaOffset=0  TranslationThetaOffsetUnits=deg  RotationMethod=StandardAxis  RotationAngleUnits=deg  RotationStandardAxis=+Y  RotationAngle=90  RotationArbitraryAxis=[0 0 1]  FollAlignAxisA=+X  BaseAlignAxisA=+Y  FollAlignAxisB=+Y  BaseAlignAxisB=+Z  RotationSequenceAxes=FollowerAxes  RotationSequence=XYX  RotationSequenceAngles=[0 0 0]  RotationSequenceAnglesUnits=deg  RotationMatrix=[1 0 0; 0 1 0; 0 0 1]  Quaternion=[1 0 0 0]
  PS-Simulink Converter : nesl_utility/PS-Simulink Converter  PhysicalDomain=network_engine_domain  SubClassName=ps_output  LeftPortType=input  RightPortType=output  PseudoPeriodic=off  Frequencies=[]  VectorFormat=inherit  Unit=inherit  AffineConversion=off
  Passive_force_norm : MATLAB Function  TreatAsAtomicUnit=on
  Simulink-PS Converter : nesl_utility/Simulink-PS Converter  PhysicalDomain=network_engine_domain  SubClassName=ps_input  LeftPortType=input  RightPortType=output  PseudoPeriodic=off  Frequencies=[]  NoiseDistribution=none  NoiseParameters=[]  Unit=1  AffineConversion=off  FilteringAndDerivatives=provide  SimscapeFilterOrder=1  InputFilterTimeConstant=0.001  UdotUserProvided=0
  Sum : Sum  Inputs=|++
  Tlak->Tah : Gain  Gain=-1
  Transform Sensor : sm_lib/Frames and Transforms/Transform Sensor  MeasurementFrame=World  RotationSequence=XYX  SenseAngle=off  SenseAxis=off  SenseQ=off  SenseR=off  SenseRotationSequence=off  SenseOmegaX=off  SenseOmegaY=off  SenseOmegaZ=off  SenseQDot=off  SenseRDot=off  SenseRotationSequenceDot=off  SenseAlphaX=off  SenseAlphaY=off  SenseAlphaZ=off  SenseQDDot=off  SenseRDDot=off  SenseX=off  SenseY=off  SenseZ=off  SenseRad=off  SenseAzim=off  SenseDist=on  SenseInc=off  SenseXDot=off  SenseYDot=off  SenseZDot=off  SenseRadDot=off  SenseAzimDot=off  SenseDistDot=off  SenseIncDot=off  SenseXDDot=off  SenseYDDot=off  SenseZDDot=off  SenseRadDDot=off  SenseAzimDDot=off  SenseDistDDot=off  SenseIncDDot=off
  l0m : Constant  Value=Glenohumeral_l0(8)
  Thorax : PMIOPort  Side=Left
  Humerus : PMIOPort  Port=2  Side=Left
  Output : Outport
  Output1 : Outport  Port=2
  wires:
  Aktivace/1 -> Active_factor_norm/3(a)
  F0M/1 -> Tlak->Tah/1
  Tlak->Tah/1 -> Output/1, Simulink-PS Converter/1
  Sum/1 -> F0M/1
  Active_factor_norm/1(Fa_norm) -> Sum/2
  Passive_force_norm/1(Fp_norm) -> Sum/1
  PS-Simulink Converter/1 -> Output1/1, Active_factor_norm/1(lm), Passive_force_norm/1(lm)
  l0m/1 -> Active_factor_norm/2(l0), Passive_force_norm/2(l0)
  connections:
  PECM1_4/RConn1 -- Internal Force1/LConn1 -- Transform Sensor/LConn1
  PECM1_3/RConn1 -- Internal Force1/RConn1 -- Transform Sensor/RConn1
  Simulink-PS Converter/RConn1 -- Internal Force1/LConn2
  PECM1_3/LConn1 -- Humerus/RConn1
  Transform Sensor/RConn2 -- PS-Simulink Converter/LConn1
  PECM1_4/LConn1 -- Thorax/RConn1

== system main/glenohumeral_muscles/SUBSC ==
  Aktivace : Inport
  Active_factor_norm : MATLAB Function  TreatAsAtomicUnit=on
  F0M : Gain  Gain=Glenohumeral_F0M(9)
  Internal Force1 : sm_lib/Forces and Torques/Internal Force
  PECM1_3 : sm_lib/Frames and Transforms/Rigid Transform  TranslationMethod=Cartesian  TranslationStandardOffset=0  TranslationStandardOffsetUnits=m  TranslationStandardAxis=+Z  TranslationCartesianOffset=[0.007 0.01 -0.023]  TranslationCartesianOffsetUnits=m  TranslationROffset=0  TranslationROffsetUnits=m  TranslationZOffset=0  TranslationZOffsetUnits=m  TranslationThetaOffset=0  TranslationThetaOffsetUnits=deg  RotationMethod=None  RotationAngleUnits=deg  RotationStandardAxis=+Z  RotationAngle=0.0  RotationArbitraryAxis=[0 0 1]  FollAlignAxisA=+X  BaseAlignAxisA=+Y  FollAlignAxisB=+Y  BaseAlignAxisB=+Z  RotationSequenceAxes=FollowerAxes  RotationSequence=XYX  RotationSequenceAngles=[0 0 0]  RotationSequenceAnglesUnits=deg  RotationMatrix=[1 0 0; 0 1 0; 0 0 1]  Quaternion=[1 0 0 0]
  PECM1_4 : sm_lib/Frames and Transforms/Rigid Transform  TranslationMethod=Cartesian  TranslationStandardOffset=0  TranslationStandardOffsetUnits=m  TranslationStandardAxis=+Z  TranslationCartesianOffset=[-0.039 -0.032 -0.033]  TranslationCartesianOffsetUnits=m  TranslationROffset=0  TranslationROffsetUnits=m  TranslationZOffset=0  TranslationZOffsetUnits=m  TranslationThetaOffset=0  TranslationThetaOffsetUnits=deg  RotationMethod=StandardAxis  RotationAngleUnits=deg  RotationStandardAxis=+Y  RotationAngle=90  RotationArbitraryAxis=[0 0 1]  FollAlignAxisA=+X  BaseAlignAxisA=+Y  FollAlignAxisB=+Y  BaseAlignAxisB=+Z  RotationSequenceAxes=FollowerAxes  RotationSequence=XYX  RotationSequenceAngles=[0 0 0]  RotationSequenceAnglesUnits=deg  RotationMatrix=[1 0 0; 0 1 0; 0 0 1]  Quaternion=[1 0 0 0]
  PS-Simulink Converter : nesl_utility/PS-Simulink Converter  PhysicalDomain=network_engine_domain  SubClassName=ps_output  LeftPortType=input  RightPortType=output  PseudoPeriodic=off  Frequencies=[]  VectorFormat=inherit  Unit=inherit  AffineConversion=off
  Passive_force_norm : MATLAB Function  TreatAsAtomicUnit=on
  Simulink-PS Converter : nesl_utility/Simulink-PS Converter  PhysicalDomain=network_engine_domain  SubClassName=ps_input  LeftPortType=input  RightPortType=output  PseudoPeriodic=off  Frequencies=[]  NoiseDistribution=none  NoiseParameters=[]  Unit=1  AffineConversion=off  FilteringAndDerivatives=provide  SimscapeFilterOrder=1  InputFilterTimeConstant=0.001  UdotUserProvided=0
  Sum : Sum  Inputs=|++
  Tlak->Tah : Gain  Gain=-1
  Transform Sensor : sm_lib/Frames and Transforms/Transform Sensor  MeasurementFrame=World  RotationSequence=XYX  SenseAngle=off  SenseAxis=off  SenseQ=off  SenseR=off  SenseRotationSequence=off  SenseOmegaX=off  SenseOmegaY=off  SenseOmegaZ=off  SenseQDot=off  SenseRDot=off  SenseRotationSequenceDot=off  SenseAlphaX=off  SenseAlphaY=off  SenseAlphaZ=off  SenseQDDot=off  SenseRDDot=off  SenseX=off  SenseY=off  SenseZ=off  SenseRad=off  SenseAzim=off  SenseDist=on  SenseInc=off  SenseXDot=off  SenseYDot=off  SenseZDot=off  SenseRadDot=off  SenseAzimDot=off  SenseDistDot=off  SenseIncDot=off  SenseXDDot=off  SenseYDDot=off  SenseZDDot=off  SenseRadDDot=off  SenseAzimDDot=off  SenseDistDDot=off  SenseIncDDot=off
  l0m : Constant  Value=Glenohumeral_l0(9)
  Scapula : PMIOPort  Side=Left
  Humerus : PMIOPort  Port=2  Side=Left
  Output : Outport
  Output1 : Outport  Port=2
  wires:
  PS-Simulink Converter/1 -> Output1/1, Active_factor_norm/1(lm), Passive_force_norm/1(lm)
  Passive_force_norm/1(Fp_norm) -> Sum/1
  Tlak->Tah/1 -> Output/1, Simulink-PS Converter/1
  Active_factor_norm/1(Fa_norm) -> Sum/2
  F0M/1 -> Tlak->Tah/1
  Sum/1 -> F0M/1
  Aktivace/1 -> Active_factor_norm/3(a)
  l0m/1 -> Active_factor_norm/2(l0), Passive_force_norm/2(l0)
  connections:
  PECM1_3/RConn1 -- Internal Force1/RConn1 -- Transform Sensor/RConn1
  PECM1_4/RConn1 -- Internal Force1/LConn1 -- Transform Sensor/LConn1
  Simulink-PS Converter/RConn1 -- Internal Force1/LConn2
  PECM1_4/LConn1 -- Scapula/RConn1
  Transform Sensor/RConn2 -- PS-Simulink Converter/LConn1
  PECM1_3/LConn1 -- Humerus/RConn1

== system main/glenohumeral_muscles/SUPSP ==
  Aktivace : Inport
  Active_factor_norm : MATLAB Function  TreatAsAtomicUnit=on
  F0M : Gain  Gain=Glenohumeral_F0M(10)
  Internal Force1 : sm_lib/Forces and Torques/Internal Force
  PECM1_3 : sm_lib/Frames and Transforms/Rigid Transform  TranslationMethod=Cartesian  TranslationStandardOffset=0  TranslationStandardOffsetUnits=m  TranslationStandardAxis=+Z  TranslationCartesianOffset=[0.04 0.031 0.006]  TranslationCartesianOffsetUnits=m  TranslationROffset=0  TranslationROffsetUnits=m  TranslationZOffset=0  TranslationZOffsetUnits=m  TranslationThetaOffset=0  TranslationThetaOffsetUnits=deg  RotationMethod=None  RotationAngleUnits=deg  RotationStandardAxis=+Z  RotationAngle=0.0  RotationArbitraryAxis=[0 0 1]  FollAlignAxisA=+X  BaseAlignAxisA=+Y  FollAlignAxisB=+Y  BaseAlignAxisB=+Z  RotationSequenceAxes=FollowerAxes  RotationSequence=XYX  RotationSequenceAngles=[0 0 0]  RotationSequenceAnglesUnits=deg  RotationMatrix=[1 0 0; 0 1 0; 0 0 1]  Quaternion=[1 0 0 0]
  PECM1_4 : sm_lib/Frames and Transforms/Rigid Transform  TranslationMethod=Cartesian  TranslationStandardOffset=0  TranslationStandardOffsetUnits=m  TranslationStandardAxis=+Z  TranslationCartesianOffset=[-0.056 -0.001 -0.041]  TranslationCartesianOffsetUnits=m  TranslationROffset=0  TranslationROffsetUnits=m  TranslationZOffset=0  TranslationZOffsetUnits=m  TranslationThetaOffset=0  TranslationThetaOffsetUnits=deg  RotationMethod=StandardAxis  RotationAngleUnits=deg  RotationStandardAxis=+Y  RotationAngle=90  RotationArbitraryAxis=[0 0 1]  FollAlignAxisA=+X  BaseAlignAxisA=+Y  FollAlignAxisB=+Y  BaseAlignAxisB=+Z  RotationSequenceAxes=FollowerAxes  RotationSequence=XYX  RotationSequenceAngles=[0 0 0]  RotationSequenceAnglesUnits=deg  RotationMatrix=[1 0 0; 0 1 0; 0 0 1]  Quaternion=[1 0 0 0]
  PS-Simulink Converter : nesl_utility/PS-Simulink Converter  PhysicalDomain=network_engine_domain  SubClassName=ps_output  LeftPortType=input  RightPortType=output  PseudoPeriodic=off  Frequencies=[]  VectorFormat=inherit  Unit=inherit  AffineConversion=off
  Passive_force_norm : MATLAB Function  TreatAsAtomicUnit=on
  Simulink-PS Converter : nesl_utility/Simulink-PS Converter  PhysicalDomain=network_engine_domain  SubClassName=ps_input  LeftPortType=input  RightPortType=output  PseudoPeriodic=off  Frequencies=[]  NoiseDistribution=none  NoiseParameters=[]  Unit=1  AffineConversion=off  FilteringAndDerivatives=provide  SimscapeFilterOrder=1  InputFilterTimeConstant=0.001  UdotUserProvided=0
  Sum : Sum  Inputs=|++
  Tlak->Tah : Gain  Gain=-1
  Transform Sensor : sm_lib/Frames and Transforms/Transform Sensor  MeasurementFrame=World  RotationSequence=XYX  SenseAngle=off  SenseAxis=off  SenseQ=off  SenseR=off  SenseRotationSequence=off  SenseOmegaX=off  SenseOmegaY=off  SenseOmegaZ=off  SenseQDot=off  SenseRDot=off  SenseRotationSequenceDot=off  SenseAlphaX=off  SenseAlphaY=off  SenseAlphaZ=off  SenseQDDot=off  SenseRDDot=off  SenseX=off  SenseY=off  SenseZ=off  SenseRad=off  SenseAzim=off  SenseDist=on  SenseInc=off  SenseXDot=off  SenseYDot=off  SenseZDot=off  SenseRadDot=off  SenseAzimDot=off  SenseDistDot=off  SenseIncDot=off  SenseXDDot=off  SenseYDDot=off  SenseZDDot=off  SenseRadDDot=off  SenseAzimDDot=off  SenseDistDDot=off  SenseIncDDot=off
  l0m : Constant  Value=Glenohumeral_l0(10)
  Scapula : PMIOPort  Side=Left
  Humerus : PMIOPort  Port=2  Side=Left
  Output : Outport
  Output1 : Outport  Port=2
  wires:
  Aktivace/1 -> Active_factor_norm/3(a)
  Sum/1 -> F0M/1
  F0M/1 -> Tlak->Tah/1
  Active_factor_norm/1(Fa_norm) -> Sum/2
  Passive_force_norm/1(Fp_norm) -> Sum/1
  l0m/1 -> Active_factor_norm/2(l0), Passive_force_norm/2(l0)
  Tlak->Tah/1 -> Output/1, Simulink-PS Converter/1
  PS-Simulink Converter/1 -> Output1/1, Active_factor_norm/1(lm), Passive_force_norm/1(lm)
  connections:
  PECM1_4/RConn1 -- Internal Force1/LConn1 -- Transform Sensor/LConn1
  PECM1_3/RConn1 -- Internal Force1/RConn1 -- Transform Sensor/RConn1
  PECM1_3/LConn1 -- Humerus/RConn1
  Transform Sensor/RConn2 -- PS-Simulink Converter/LConn1
  Simulink-PS Converter/RConn1 -- Internal Force1/LConn2
  PECM1_4/LConn1 -- Scapula/RConn1

== system main/glenohumeral_muscles/TMAJ ==
  Aktivace : Inport
  Active_factor_norm : MATLAB Function  TreatAsAtomicUnit=on
  F0M : Gain  Gain=Glenohumeral_F0M(11)
  Internal Force1 : sm_lib/Forces and Torques/Internal Force
  PECM1_3 : sm_lib/Frames and Transforms/Rigid Transform  TranslationMethod=Cartesian  TranslationStandardOffset=0  TranslationStandardOffsetUnits=m  TranslationStandardAxis=+Z  TranslationCartesianOffset=[0.004 -0.045 -0.007]  TranslationCartesianOffsetUnits=m  TranslationROffset=0  TranslationROffsetUnits=m  TranslationZOffset=0  TranslationZOffsetUnits=m  TranslationThetaOffset=0  TranslationThetaOffsetUnits=deg  RotationMethod=None  RotationAngleUnits=deg  RotationStandardAxis=+Z  RotationAngle=0.0  RotationArbitraryAxis=[0 0 1]  FollAlignAxisA=+X  BaseAlignAxisA=+Y  FollAlignAxisB=+Y  BaseAlignAxisB=+Z  RotationSequenceAxes=FollowerAxes  RotationSequence=XYX  RotationSequenceAngles=[0 0 0]  RotationSequenceAnglesUnits=deg  RotationMatrix=[1 0 0; 0 1 0; 0 0 1]  Quaternion=[1 0 0 0]
  PECM1_4 : sm_lib/Frames and Transforms/Rigid Transform  TranslationMethod=Cartesian  TranslationStandardOffset=0  TranslationStandardOffsetUnits=m  TranslationStandardAxis=+Z  TranslationCartesianOffset=[-0.045 -0.106 -0.002]  TranslationCartesianOffsetUnits=m  TranslationROffset=0  TranslationROffsetUnits=m  TranslationZOffset=0  TranslationZOffsetUnits=m  TranslationThetaOffset=0  TranslationThetaOffsetUnits=deg  RotationMethod=StandardAxis  RotationAngleUnits=deg  RotationStandardAxis=+Y  RotationAngle=90  RotationArbitraryAxis=[0 0 1]  FollAlignAxisA=+X  BaseAlignAxisA=+Y  FollAlignAxisB=+Y  BaseAlignAxisB=+Z  RotationSequenceAxes=FollowerAxes  RotationSequence=XYX  RotationSequenceAngles=[0 0 0]  RotationSequenceAnglesUnits=deg  RotationMatrix=[1 0 0; 0 1 0; 0 0 1]  Quaternion=[1 0 0 0]
  PS-Simulink Converter : nesl_utility/PS-Simulink Converter  PhysicalDomain=network_engine_domain  SubClassName=ps_output  LeftPortType=input  RightPortType=output  PseudoPeriodic=off  Frequencies=[]  VectorFormat=inherit  Unit=inherit  AffineConversion=off
  Passive_force_norm : MATLAB Function  TreatAsAtomicUnit=on
  Simulink-PS Converter : nesl_utility/Simulink-PS Converter  PhysicalDomain=network_engine_domain  SubClassName=ps_input  LeftPortType=input  RightPortType=output  PseudoPeriodic=off  Frequencies=[]  NoiseDistribution=none  NoiseParameters=[]  Unit=1  AffineConversion=off  FilteringAndDerivatives=provide  SimscapeFilterOrder=1  InputFilterTimeConstant=0.001  UdotUserProvided=0
  Sum : Sum  Inputs=|++
  Tlak->Tah : Gain  Gain=-1
  Transform Sensor : sm_lib/Frames and Transforms/Transform Sensor  MeasurementFrame=World  RotationSequence=XYX  SenseAngle=off  SenseAxis=off  SenseQ=off  SenseR=off  SenseRotationSequence=off  SenseOmegaX=off  SenseOmegaY=off  SenseOmegaZ=off  SenseQDot=off  SenseRDot=off  SenseRotationSequenceDot=off  SenseAlphaX=off  SenseAlphaY=off  SenseAlphaZ=off  SenseQDDot=off  SenseRDDot=off  SenseX=off  SenseY=off  SenseZ=off  SenseRad=off  SenseAzim=off  SenseDist=on  SenseInc=off  SenseXDot=off  SenseYDot=off  SenseZDot=off  SenseRadDot=off  SenseAzimDot=off  SenseDistDot=off  SenseIncDot=off  SenseXDDot=off  SenseYDDot=off  SenseZDDot=off  SenseRadDDot=off  SenseAzimDDot=off  SenseDistDDot=off  SenseIncDDot=off
  l0m : Constant  Value=Glenohumeral_l0(11)
  Scapula : PMIOPort  Side=Left
  Humerus : PMIOPort  Port=2  Side=Left
  Output : Outport
  Output1 : Outport  Port=2
  wires:
  l0m/1 -> Active_factor_norm/2(l0), Passive_force_norm/2(l0)
  Active_factor_norm/1(Fa_norm) -> Sum/2
  Sum/1 -> F0M/1
  Aktivace/1 -> Active_factor_norm/3(a)
  Passive_force_norm/1(Fp_norm) -> Sum/1
  Tlak->Tah/1 -> Output/1, Simulink-PS Converter/1
  F0M/1 -> Tlak->Tah/1
  PS-Simulink Converter/1 -> Output1/1, Active_factor_norm/1(lm), Passive_force_norm/1(lm)
  connections:
  PECM1_4/RConn1 -- Internal Force1/LConn1 -- Transform Sensor/LConn1
  PECM1_3/RConn1 -- Internal Force1/RConn1 -- Transform Sensor/RConn1
  PECM1_3/LConn1 -- Humerus/RConn1
  Simulink-PS Converter/RConn1 -- Internal Force1/LConn2
  Transform Sensor/RConn2 -- PS-Simulink Converter/LConn1
  PECM1_4/LConn1 -- Scapula/RConn1
